simulink model "BEV_Laengsdynamikmodell_v2"  (R2024a)
settings: configuration reference "SharedConfig" (kept outside this file)
values from neighbouring files (symbols this model uses):
  acc_cycle_flag = 0    [simulink_function_handle_v2.m]
  battery = sim_BTMS_interface(battery,config_battery, config_vehicle)    [init_simulation.m]    (also in simulink_function_handle_v2.m = evalin('base', 'battery'))
  config_battery = read_json_config("config/conf_battery.json")    [Sim_v2.m]    (also in init_simulation.m = evalin('base', 'config_battery'); simulink_function_handle_v2.m = cell_loader(config_battery, bat_cell_capacity, bat_celltype )
  config_gearbox = evalin("base", "config_gearbox")    [simulink_function_handle_v2.m]
  config_Inverter = read_json_config("config/conf_Inverter.json")    [Sim_v2.m]
  config_motor = evalin("base","config_motor")    [simulink_function_handle_v2.m]
  config_vehicle = read_json_config(vehicle_config_file)    [Sim_v2.m]    (also in import_dc_cycle.m = evalin('base', 'config_vehicle'); init_simulation.m = evalin('base', 'config_vehicle'); simulink_function_handle_v2.m = evalin('base','config_vehicle'))
  k_FW = 410/(14e3)^2.5    (= 1.76792471652e-08)    [simulink_function_handle_v2.m]
  ModuleType1 = evalin("base","ModuleType1")    [simulink_function_handle_v2.m]
undefined symbols (not defined in the file or in its folder): Analyse, battery_builder_rtmsupport, GB, gcbh, gearbox_map, ModuleAssembly1, motormap
libraries: spsParallelRLCBranchLib x20, nesl_utility x18, GD_Batterymodel_NSGAII_1_lib x12, BatteryProtection x9, spsControlledCurrentSourceLib x8, spsVoltageMeasurementLib x8, fl_lib x7, dspstat3 x4, spsDCVoltageSourceLib x4, spspowerguiLib x4, simulink x3, eePmsmCurrentReferenceGen x2
(part 2 of 5)

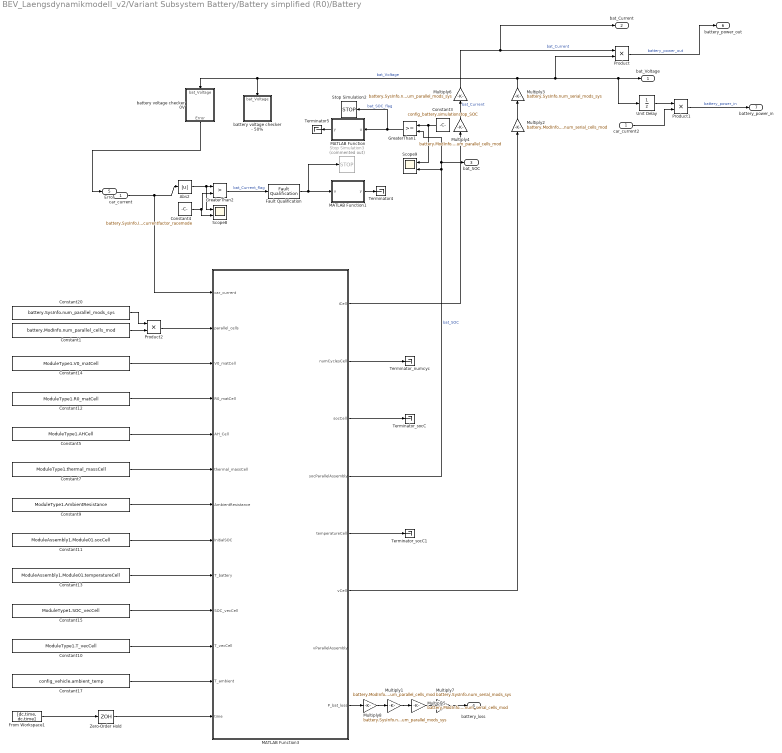
== system BEV_Laengsdynamikmodell_v2/Variant Subsystem Battery/Battery simplified (R0)/Battery ==
  car_current : Inport
  Abs2 : Abs  SaturateOnIntegerOverflow=off
  Constant1 : Constant  Value=battery.ModInfo.num_parallel_cells_mod
  Constant10 : Constant  Value=ModuleType1.T_vecCell
  Constant11 : Constant  Value=ModuleAssembly1.Module01.socCell
  Constant12 : Constant  Value=ModuleType1.R0_matCell
  Constant13 : Constant  Value=ModuleAssembly1.Module01.temperatureCell
  Constant14 : Constant  Value=ModuleType1.V0_matCell
  Constant15 : Constant  Value=ModuleType1.SOC_vecCell
  Constant17 : Constant  Value=config_vehicle.ambient_temp
  Constant20 : Constant  Value=battery.SysInfo.num_parallel_mods_sys
  Constant3 : Constant  Value=config_battery.simulationstop_SOC
  Constant4 : Constant  Value=battery.SysInfo.I_max_sys * config_battery.overcurrentfactor_racemode
  Constant5 : Constant  Value=ModuleType1.AHCell
  Constant7 : Constant  Value=ModuleType1.thermal_massCell
  Constant9 : Constant  Value=ModuleType1.AmbientResistance
  Fault Qualification : BatteryProtection/Fault Qualification  QualTime=3  DisqualTime=6  Ts=-1
      settings: LibrarySourceBlock=batt_sl_lib/Protection/Fault Qualification
  From Workspace1 : FromWorkspace  VariableName=[dc.time, dc.time]
  GreaterThan1 : RelationalOperator  OutDataTypeStr=boolean  RndMeth=Simplest  InputSameDT=off
  GreaterThan2 : RelationalOperator  Operator=>  OutDataTypeStr=boolean  RndMeth=Simplest  InputSameDT=off
  MATLAB Function : MATLAB Function  TreatAsAtomicUnit=on
  MATLAB Function1 : MATLAB Function  TreatAsAtomicUnit=on
  MATLAB Function3 : MATLAB Function  TreatAsAtomicUnit=on
  Multiply1 : Gain  Gain=battery.ModInfo.num_parallel_cells_mod
  Multiply2 : Gain  Gain=battery.ModInfo.num_serial_cells_mod
  Multiply3 : Gain  Gain=battery.SysInfo.num_serial_mods_sys
  Multiply4 : Gain  Gain=battery.ModInfo.num_parallel_cells_mod
  Multiply5 : Gain  Gain=battery.ModInfo.num_serial_cells_mod
  Multiply6 : Gain  Gain=battery.SysInfo.num_parallel_mods_sys
  Multiply7 : Gain  Gain=battery.SysInfo.num_serial_mods_sys
  Multiply8 : Gain  Gain=battery.SysInfo.num_parallel_mods_sys
  Product : Product
  Product1 : Product
  Product2 : Product
  Scope8 : Scope  NumInputPorts=2
  Scope9 : Scope  NumInputPorts=2
  Stop Simulation2 : Stop
  Stop Simulation3 : Stop  Commented=on
  Terminator4 : Terminator
  Terminator5 : Terminator
  Terminator_numcyc : Terminator
  Terminator_socC : Terminator
  Terminator_socC1 : Terminator
  Unit Delay : UnitDelay  SampleTime=-1  HasFrameUpgradeWarning=on
  Zero-Order Hold : ZeroOrderHold  SampleTime=-1
  battery voltage checker - 50% : Subsystem
  battery voltage checker 0V : Subsystem
  car_current2 : InportShadow
  bat_Voltage : Outport
  bat_Current : Outport  Port=2
  bat_SOC : Outport  Port=3
  battery_loss : Outport  Port=4
  Error : Outport  Port=5
  battery_power_out : Outport  Port=6
  battery_power_in : Outport  Port=7
  wires:
  Constant3/1 -> GreaterThan1/1, Scope9/1
  car_current/1 -> MATLAB Function3/1(car_current), Abs2/1
  MATLAB Function3/6(vCell) -> Multiply2/1
  Multiply3/1 -> Product/2, bat_Voltage/1, Unit Delay/1, battery voltage checker - 50%/1(bat_Voltage), battery voltage checker 0V/1(bat_Voltage)  "bat_Voltage"
  Abs2/1 -> Scope8/1, GreaterThan2/1
  Constant4/1 -> Scope8/2, GreaterThan2/2
  MATLAB Function3/4(socParallelAssembly) -> GreaterThan1/2, bat_SOC/1, Scope9/2  "bat_SOC"
  MATLAB Function3/1(iCell) -> Multiply4/1
  GreaterThan1/1 -> Stop Simulation2/1, MATLAB Function/1(u)  "bat_SOC_flag"
  GreaterThan2/1 -> Fault Qualification/1  "bat_Current_flag"
  MATLAB Function/1(y) -> Terminator5/1
  MATLAB Function1/1(y) -> Terminator4/1
  Multiply4/1 -> Multiply6/1  "bat_Current"
  MATLAB Function3/3(socCell) -> Terminator_socC/1
  battery voltage checker 0V/1(Error) -> Error/1
  Multiply2/1 -> Multiply3/1
  Fault Qualification/1 -> Stop Simulation3/1, MATLAB Function1/1(u)
  MATLAB Function3/2(numCyclesCell) -> Terminator_numcyc/1
  MATLAB Function3/5(temperatureCell) -> Terminator_socC1/1
  car_current2/1 -> Product1/2
  Unit Delay/1 -> Product1/1
  Multiply6/1 -> bat_Current/1, Product/1  "bat_Current"
  Product1/1 -> battery_power_in/1  "battery_power_in"
  Product/1 -> battery_power_out/1  "battery_power_out"
  Zero-Order Hold/1 -> MATLAB Function3/13(time)
  From Workspace1/1 -> Zero-Order Hold/1
  Constant5/1 -> MATLAB Function3/5(AH_Cell)
  Constant13/1 -> MATLAB Function3/9(T_battery)
  Constant11/1 -> MATLAB Function3/8(InitialSOC)
  Constant14/1 -> MATLAB Function3/3(V0_matCell)
  Constant12/1 -> MATLAB Function3/4(R0_matCell)
  Constant15/1 -> MATLAB Function3/10(SOC_vecCell)
  Constant7/1 -> MATLAB Function3/6(thermal_massCell)
  Constant10/1 -> MATLAB Function3/11(T_vecCell)
  Constant9/1 -> MATLAB Function3/7(AmbientResistance)
  Constant17/1 -> MATLAB Function3/12(T_ambient)
  Multiply7/1 -> battery_loss/1
  MATLAB Function3/8(P_bat_loss) -> Multiply8/1
  Multiply5/1 -> Multiply7/1
  Multiply1/1 -> Multiply5/1
  Constant1/1 -> Product2/2
  Constant20/1 -> Product2/1
  Product2/1 -> MATLAB Function3/2(parallel_cells)
  Multiply8/1 -> Multiply1/1

== system BEV_Laengsdynamikmodell_v2/Variant Subsystem Gearbox/Gearbox Analytic/Oil Temp ==
  P_V : Inport
  IC : InitialCondition  Value=25
  MATLAB Function : MATLAB Function  TreatAsAtomicUnit=on
  Memory1 : Memory  InitialCondition=config_vehicle.ambient_temp - 273
  Memory2 : Memory  InitialCondition=config_vehicle.ambient_temp - 273
  Scope : Scope
  temp : Outport
  wires:
  MATLAB Function/1(T) -> IC/1  "GB_temp"
  Memory1/1 -> MATLAB Function/1(t)
  P_V/1 -> Memory2/1
  IC/1 -> Scope/1, Memory1/1, temp/1
  Memory2/1 -> MATLAB Function/2(P_V)

== system BEV_Laengsdynamikmodell_v2/Variant Subsystem Gearbox/Gearbox Analytic/Oil Temp Gao ==
  note: entspricht 2pi/60 * 1e-3
  T_wheel : Inport
  rpm_wheel : Inport  Port=2
  MATLAB Function : MATLAB Function  TreatAsAtomicUnit=on
  Memory1 : Memory  InitialCondition=config_vehicle.ambient_temp - 273
  Multiply5 : Gain  Gain=1/9550
  Product2 : Product
  Scope : Scope
  temp : Outport
  wires:
  Product2/1 -> Multiply5/1
  rpm_wheel/1 -> MATLAB Function/3(rpm), Product2/2
  T_wheel/1 -> Product2/1
  MATLAB Function/1(T) -> Scope/1, Memory1/1, temp/1
  Memory1/1 -> MATLAB Function/1(t)
  Multiply5/1 -> MATLAB Function/2(P)

== system BEV_Laengsdynamikmodell_v2/Variant Subsystem Gearbox/Gearbox Analytic/Variant Subsystem Analytic GB ==
  note: 1) Add Subsystem or Model blocks as valid variant choices.
      | 2) You cannot connect blocks at this level. At simulation, connectivity is automatically
      | determined, based on the active variant and port name matching.
  wheel_torque : Inport
  wheel_rpm : Inport  Port=2
  Temp : Inport  Port=3
  Einstufig_Achsparallel : Subsystem  VariantControl=GB_Stufen == 1
  Zweistufig_Achsparallel : Subsystem  VariantControl="GB_Stufen == 2 && GB_Topology == \"achsparallel\""
  Zweistufig_Koaxial : Subsystem  VariantControl="GB_Stufen == 2 && GB_Topology == \"koaxial\""
  P_V : Outport

== system BEV_Laengsdynamikmodell_v2/Variant Subsystem Gearbox/Gearbox Lookup-Table/Oil Temp ==
  P_V : Inport
  IC : InitialCondition  Value=25
  MATLAB Function : MATLAB Function  TreatAsAtomicUnit=on
  Memory1 : Memory  InitialCondition=config_vehicle.ambient_temp - 273
  Memory2 : Memory  InitialCondition=config_vehicle.ambient_temp - 273
  Scope : Scope
  temp : Outport
  wires:
  MATLAB Function/1(T) -> IC/1  "GB_temp"
  Memory1/1 -> MATLAB Function/1(t)
  P_V/1 -> Memory2/1
  IC/1 -> Scope/1, Memory1/1, temp/1
  Memory2/1 -> MATLAB Function/2(P_V)

== system BEV_Laengsdynamikmodell_v2/Variant Subsystem Gearbox/Gearbox Lookup-Table/Oil Temp Gao ==
  note: entspricht 2pi/60 * 1e-3
  T_wheel : Inport
  rpm_wheel : Inport  Port=2
  MATLAB Function : MATLAB Function  TreatAsAtomicUnit=on
  Memory1 : Memory  InitialCondition=config_vehicle.ambient_temp - 273
  Multiply5 : Gain  Gain=1/9550
  Product2 : Product
  Scope : Scope
  temp : Outport
  wires:
  Product2/1 -> Multiply5/1
  rpm_wheel/1 -> MATLAB Function/3(rpm), Product2/2
  T_wheel/1 -> Product2/1
  MATLAB Function/1(T) -> Scope/1, Memory1/1, temp/1
  Memory1/1 -> MATLAB Function/1(t)
  Multiply5/1 -> MATLAB Function/2(P)

== system BEV_Laengsdynamikmodell_v2/Variant Subsystem Gearbox/Gearbox Lookup-Table/Variant Subsystem ==
  note: 1) Add Subsystem or Model blocks as valid variant choices.
      | 2) You cannot connect blocks at this level. At simulation, connectivity is automatically
      | determined, based on the active variant and port name matching.
  wheel_torque : Inport
  wheel_rpm : Inport  Port=2
  Temp : Inport  Port=3
  ETA_map : Subsystem  VariantControl="gearbox_map.map_type == \"Eta\""
  LOSS_map : Subsystem  VariantControl="gearbox_map.map_type == \"Loss\""
  loss_lockup : Outport
  gearbox_efficiency : Outport  Port=2
  gearbox_rpm : Outport  Port=3
  gearbox_torque : Outport  Port=4

== system BEV_Laengsdynamikmodell_v2/Variant Subsystem Inverter/Inverter Analytic/Variant Subsystem ==
  note: 1) Add Subsystem or Model blocks as valid variant choices.
      | 2) You cannot connect blocks at this level. At simulation, connectivity is automatically
      | determined, based on the active variant and port name matching.
  udc : Inport
  rpm : Inport  Port=2
  torque : Inport  Port=3
  terminal_power : Inport  Port=4
  IM_Inverter_IGBT_Analytic : Subsystem  VariantControl=Mode_IM_IGBT
  IM_Inverter_SiC-MOSFET_Analytic : Subsystem  VariantControl=Mode_IM_MOSFET
  PMSM_Inverter_IBGT_Analytic : Subsystem  VariantControl=Mode_PSM_IGBT
  PMSM_Inverter_SiC-MOSFET_Analytic : Subsystem  VariantControl=Mode_PSM_MOSFET
  Conduction_and_Switching_loss : Outport
  idc : Outport  Port=2
  P_inv_total : Outport  Port=3
  P_mot_elec : Outport  Port=4

== system BEV_Laengsdynamikmodell_v2/Variant Subsystem Motor/Motor Analytic/Friction & Windage ==
  note: Gleichung für mechanische Verlustleistung:
      | P_FW = k_FW * n^2.5
  gearbox_rpm : Inport
  Constant : Constant  Value=2.5
  Constant1 : Constant  Value=0
  Constant5 : Constant  Value=k_FW
  Gain : Gain  Gain=2*pi/60
  In2 : InportShadow
  Power : Math  Operator=pow
  Product : Product
  Product2 : Product  Inputs=*/
  Switch : Switch  Criteria=u2 > Threshold  SaturateOnIntegerOverflow=off  InputSameDT=off
  friction torque : Outport
  wires:
  gearbox_rpm/1 -> Power/1  "n_gearbox"
  Constant/1 -> Power/2  "exponent"
  Power/1 -> Product/1
  Constant5/1 -> Product/2
  Product/1 -> Product2/1  "mech powerloss"
  Product2/1 -> Switch/1  "torque"
  In2/1 -> Gain/1  "n_gearbox"
  Gain/1 -> Product2/2, Switch/2
  Switch/1 -> friction torque/1
  Constant1/1 -> Switch/3

== system BEV_Laengsdynamikmodell_v2/Variant Subsystem Motor/Motor Const/Friction & Windage ==
  note: Gleichung für mechanische Verlustleistung:
      | P_FW = k_FW * n^2.5
  gearbox_rpm : Inport
  Constant : Constant  Value=2.5
  Constant1 : Constant  Value=0
  Constant5 : Constant  Value=k_FW
  Gain : Gain  Gain=2*pi/60
  In2 : InportShadow
  Power : Math  Operator=pow
  Product : Product
  Product2 : Product  Inputs=*/
  Switch : Switch  Criteria=u2 > Threshold  SaturateOnIntegerOverflow=off  InputSameDT=off
  friction torque : Outport
  wires:
  gearbox_rpm/1 -> Power/1  "n_gearbox"
  Constant/1 -> Power/2  "exponent"
  Power/1 -> Product/1
  Constant5/1 -> Product/2
  Product/1 -> Product2/1  "mech powerloss"
  Product2/1 -> Switch/1  "torque"
  In2/1 -> Gain/1  "n_gearbox"
  Gain/1 -> Product2/2, Switch/2
  Switch/1 -> friction torque/1
  Constant1/1 -> Switch/3

== system BEV_Laengsdynamikmodell_v2/Variant Subsystem Motor/Motor Lookup-Table/Friction & Windage ==
  note: Gleichung für mechanische Verlustleistung:
      | P_FW = k_FW * n^2.5
  gearbox_rpm : Inport
  Constant : Constant  Value=2.5
  Constant1 : Constant  Value=0
  Constant5 : Constant  Value=k_FW
  Gain : Gain  Gain=2*pi/60
  In2 : InportShadow
  Power : Math  Operator=pow
  Product : Product
  Product2 : Product  Inputs=*/
  Switch : Switch  Criteria=u2 > Threshold  SaturateOnIntegerOverflow=off  InputSameDT=off
  friction torque : Outport
  wires:
  gearbox_rpm/1 -> Power/1  "n_gearbox"
  Constant/1 -> Power/2  "exponent"
  Power/1 -> Product/1
  Constant5/1 -> Product/2
  Product/1 -> Product2/1  "mech powerloss"
  Product2/1 -> Switch/1  "torque"
  In2/1 -> Gain/1  "n_gearbox"
  Gain/1 -> Product2/2, Switch/2
  Switch/1 -> friction torque/1
  Constant1/1 -> Switch/3

== system BEV_Laengsdynamikmodell_v2/Variant Subsystem Battery/Battery Analytic (RC3)/Battery/battery voltage checker - 50% ==
  bat_Voltage : Inport
  Constant : Constant  Value=acc_cycle_flag
  Constant5 : Constant  Value=0.5 * battery.SysInfo.U_max_sys
  Data Type Conversion : DataTypeConversion  OutDataTypeStr=double  SaturateOnIntegerOverflow=off  RndMeth=Floor
  Fault Qualification : BatteryProtection/Fault Qualification  QualTime=2  DisqualTime=4  Ts=-1
      settings: LibrarySourceBlock=batt_sl_lib/Protection/Fault Qualification
  GreaterThan3 : RelationalOperator  Operator=>  OutDataTypeStr=boolean  RndMeth=Simplest  InputSameDT=off
  MATLAB Function2 : MATLAB Function  TreatAsAtomicUnit=on
  Stop Simulation : Stop
  Unit Delay : UnitDelay  SampleTime=-1  HasFrameUpgradeWarning=on
  wires:
  Constant/1 -> MATLAB Function2/3(z)
  Fault Qualification/1 -> MATLAB Function2/1(u)
  MATLAB Function2/2(st) -> Stop Simulation/1
  Data Type Conversion/1 -> MATLAB Function2/2(d)
  Unit Delay/1 -> Data Type Conversion/1
  MATLAB Function2/1(y) -> Unit Delay/1
  bat_Voltage/1 -> GreaterThan3/2
  GreaterThan3/1 -> Fault Qualification/1
  Constant5/1 -> GreaterThan3/1

== system BEV_Laengsdynamikmodell_v2/Variant Subsystem Battery/Battery Analytic (RC3)/Battery/battery voltage checker 0V ==
  bat_Voltage : Inport
  Constant7 : Constant  Value=0
  Fault Qualification1 : BatteryProtection/Fault Qualification  QualTime=1  DisqualTime=3  Ts=-1
      settings: LibrarySourceBlock=batt_sl_lib/Protection/Fault Qualification
  GreaterThan4 : RelationalOperator  Operator=>  OutDataTypeStr=boolean  RndMeth=Simplest  InputSameDT=off
  Error : Outport
  wires:
  Fault Qualification1/1 -> Error/1
  bat_Voltage/1 -> GreaterThan4/2
  GreaterThan4/1 -> Fault Qualification1/1
  Constant7/1 -> GreaterThan4/1

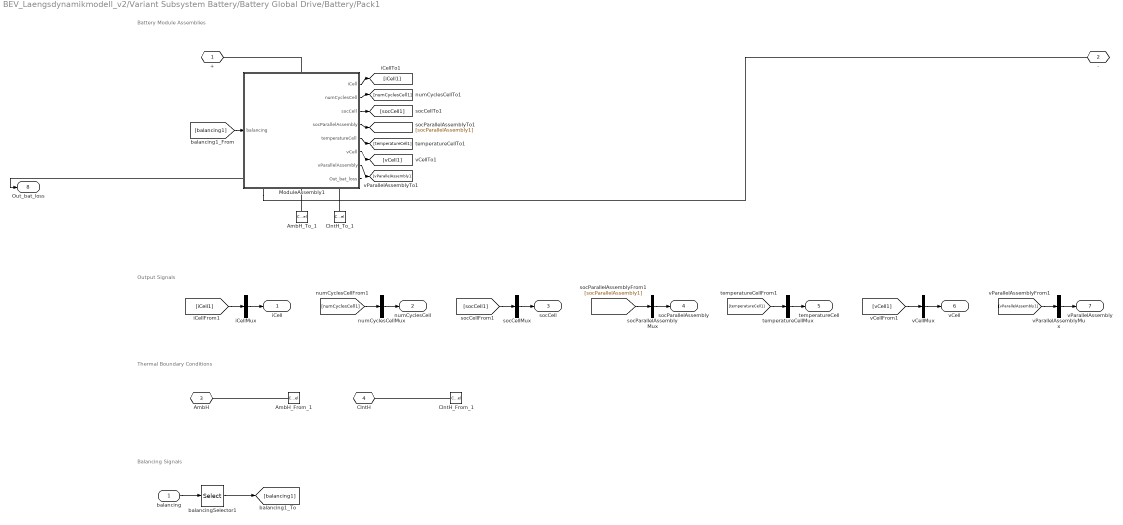
== system BEV_Laengsdynamikmodell_v2/Variant Subsystem Battery/Battery Global Drive/Battery/Pack1 ==
  note: Balancing Signals
  note: Thermal Boundary Conditions
  note: Output Signals
  note: Battery Module Assemblies
  balancing : Inport  PortDimensions=120
  AmbH_From_1 : ConnectionLabel  Label=ambH_1
  AmbH_To_1 : ConnectionLabel  Label=ambH_1
  ClntH_From_1 : ConnectionLabel  Label=clntH_1
  ClntH_To_1 : ConnectionLabel  Label=clntH_1
  ModuleAssembly1 : Subsystem  LoadFcn=battery_builder_rtmsupport('loadfcn',gcbh);
      settings: CopyFcn=battery_builder_rtmsupport('copyfcn',gcbh);  PreCopyFcn=battery_builder_rtmsupport('precopyfcn',gcbh);  PreDeleteFcn=battery_builder_rtmsupport('predeletefcn',gcbh);  PortSchema="{\"entries\":[{\"content\":{\"sides\":[{\"content\":{\"connectorIds\":[\"LConn1\"]},\"type\":\"ConnectorPlacement.EquallySpacedRectSide\",\"uuid\":\"39e93321-efac-446f-a75c-eda4d8d6b0d6\"},{\"content\":{\"connectorIds\":[\"RConn1\",\"RConn2\",\"RConn3\"],\"side\":\"RIGHT\"},\"type\":\"ConnectorPlacement.EquallySpacedRectSide\",\"uuid\":\"10ad7812-c6c9-4cb3-b6be-c67a3fc87af4\"},{\"content\":{\"connectorIds\":[\"In1\"],\"side\":\"TOP\"},\"type\":\"ConnectorPlacement.EquallySpacedRectSide\",\"uuid\":\"ea32dac7-a4ac-4f16-bcf8-bfac99073aa1\"},{\"content\":{\"connectorIds\":[\"Out1\",\"Out2\",\"Out3\",\"Out4\",\"Out5\",\"Out6\",\"Out7\",\"Out8\"],\"side\":\"BOTTOM\"},\"type\":\"ConnectorPlacement.EquallySpacedRectSide\",\"uuid\":\"2a45af1c-2d64-4e86-8177-57e80a443e25\"}]},\"type\":\"ConnectorPlacement.EquallySpacedConnector\",\"uuid\":\"ff988f0c-c525-4dd2-8156-8cb001cdab44\"}],\"packageUris\":[\"http://schema.mathworks.com/mf0/Connector/R2020b\"],\"version\":\"1.0\"}"
      mask Display: image('$imagefile')
  balancingSelector1 : Selector  InputPortWidth=120  IndexOptions=Index vector (dialog)  Indices="[1    2    3    4    5    6    7    8    9   10   11   12   13   14   15   16   17   18   19   20   21   22   23   24   25   26   27   28   29   30   31   32   33   34   35   36   37   38   39   40   41   42   43   44   45   46   47   48   49   50   51   52   53   54   55   56   57   58   59   60   61   62   63   64   65   66   67   68   69   70   71   72   73   74   75   76   77   78   79   80   81   82   83   84   85   86   87   88   89   90   91   92   93   94   95   96   97   98   99  100  101  102  103  104  105  106  107  108  109  110  111  112  113  114  115  116  117  118  119  120]"  OutputSizes=1
  iCellMux : Mux  Inputs=1
  numCyclesCellMux : Mux  Inputs=1
  socCellMux : Mux  Inputs=1
  socParallelAssemblyMux : Mux  Inputs=1
  temperatureCellMux : Mux  Inputs=1
  vCellMux : Mux  Inputs=1
  vParallelAssemblyMux : Mux  Inputs=1
  + : PMIOPort  Side=Left
  - : PMIOPort  Port=2  Side=Right
  AmbH : PMIOPort  Port=3  Side=Right  ConnectionType=Connection: foundation.thermal.thermal
  ClntH : PMIOPort  Port=4  Side=Right  ConnectionType=Connection: foundation.thermal.thermal
  iCell : Outport
  numCyclesCell : Outport  Port=2
  socCell : Outport  Port=3
  socParallelAssembly : Outport  Port=4
  temperatureCell : Outport  Port=5
  vCell : Outport  Port=6
  vParallelAssembly : Outport  Port=7
  Out_bat_loss : Outport  Port=8
  wires:
  balancingSelector1/1 -> [balancing1]
  balancing/1 -> balancingSelector1/1
  [balancing1] -> ModuleAssembly1/1(balancing)
  [vParallelAssembly1] -> vParallelAssemblyMux/1
  vParallelAssemblyMux/1 -> vParallelAssembly/1
  ModuleAssembly1/7(vParallelAssembly) -> [vParallelAssembly1]
  [vCell1] -> vCellMux/1
  vCellMux/1 -> vCell/1
  ModuleAssembly1/6(vCell) -> [vCell1]
  [temperatureCell1] -> temperatureCellMux/1
  temperatureCellMux/1 -> temperatureCell/1
  ModuleAssembly1/5(temperatureCell) -> [temperatureCell1]
  [socParallelAssembly1] -> socParallelAssemblyMux/1
  socParallelAssemblyMux/1 -> socParallelAssembly/1
  ModuleAssembly1/4(socParallelAssembly) -> [socParallelAssembly1]
  [socCell1] -> socCellMux/1
  socCellMux/1 -> socCell/1
  ModuleAssembly1/3(socCell) -> [socCell1]
  [numCyclesCell1] -> numCyclesCellMux/1
  numCyclesCellMux/1 -> numCyclesCell/1
  ModuleAssembly1/2(numCyclesCell) -> [numCyclesCell1]
  [iCell1] -> iCellMux/1
  iCellMux/1 -> iCell/1
  ModuleAssembly1/1(iCell) -> [iCell1]
  ModuleAssembly1/8(Out_bat_loss) -> Out_bat_loss/1
  connections:
  ClntH_From_1/LConn1 -- ClntH/RConn1
  ClntH_To_1/LConn1 -- ModuleAssembly1/RConn3
  AmbH_From_1/LConn1 -- AmbH/RConn1
  AmbH_To_1/LConn1 -- ModuleAssembly1/RConn2
  ModuleAssembly1/RConn1 -- -/RConn1
  ModuleAssembly1/LConn1 -- +/RConn1

== system BEV_Laengsdynamikmodell_v2/Variant Subsystem Battery/Battery Global Drive/Battery/battery voltage checker - 50% ==
  bat_Voltage : Inport
  Constant : Constant  Value=acc_cycle_flag
  Constant5 : Constant  Value=0.5 * battery.SysInfo.U_max_sys
  Data Type Conversion : DataTypeConversion  OutDataTypeStr=double  SaturateOnIntegerOverflow=off  RndMeth=Floor
  Fault Qualification : BatteryProtection/Fault Qualification  QualTime=2  DisqualTime=4  Ts=-1
      settings: LibrarySourceBlock=batt_sl_lib/Protection/Fault Qualification
  GreaterThan3 : RelationalOperator  Operator=>  OutDataTypeStr=boolean  RndMeth=Simplest  InputSameDT=off
  MATLAB Function2 : MATLAB Function  TreatAsAtomicUnit=on
  Stop Simulation : Stop
  Unit Delay : UnitDelay  SampleTime=-1  HasFrameUpgradeWarning=on
  wires:
  Constant5/1 -> GreaterThan3/1
  GreaterThan3/1 -> Fault Qualification/1
  bat_Voltage/1 -> GreaterThan3/2
  MATLAB Function2/1(y) -> Unit Delay/1
  Unit Delay/1 -> Data Type Conversion/1
  Data Type Conversion/1 -> MATLAB Function2/2(d)
  MATLAB Function2/2(st) -> Stop Simulation/1
  Fault Qualification/1 -> MATLAB Function2/1(u)
  Constant/1 -> MATLAB Function2/3(z)

== system BEV_Laengsdynamikmodell_v2/Variant Subsystem Battery/Battery Global Drive/Battery/battery voltage checker 0V ==
  bat_Voltage : Inport
  Constant7 : Constant  Value=0
  Fault Qualification1 : BatteryProtection/Fault Qualification  QualTime=1  DisqualTime=3  Ts=-1
      settings: LibrarySourceBlock=batt_sl_lib/Protection/Fault Qualification
  GreaterThan4 : RelationalOperator  Operator=>  OutDataTypeStr=boolean  RndMeth=Simplest  InputSameDT=off
  Error : Outport
  wires:
  Constant7/1 -> GreaterThan4/1
  GreaterThan4/1 -> Fault Qualification1/1
  bat_Voltage/1 -> GreaterThan4/2
  Fault Qualification1/1 -> Error/1

== system BEV_Laengsdynamikmodell_v2/Variant Subsystem Battery/Battery simplified (R0)/Battery/battery voltage checker - 50% ==
  bat_Voltage : Inport
  Constant : Constant  Value=acc_cycle_flag
  Constant5 : Constant  Value=0.5 * battery.SysInfo.U_max_sys
  Data Type Conversion : DataTypeConversion  OutDataTypeStr=double  SaturateOnIntegerOverflow=off  RndMeth=Floor
  Fault Qualification : BatteryProtection/Fault Qualification  QualTime=2  DisqualTime=4  Ts=-1
      settings: LibrarySourceBlock=batt_sl_lib/Protection/Fault Qualification
  GreaterThan3 : RelationalOperator  Operator=>  OutDataTypeStr=boolean  RndMeth=Simplest  InputSameDT=off
  MATLAB Function2 : MATLAB Function  TreatAsAtomicUnit=on
  Stop Simulation : Stop
  Unit Delay : UnitDelay  SampleTime=-1  HasFrameUpgradeWarning=on
  wires:
  Constant5/1 -> GreaterThan3/1
  GreaterThan3/1 -> Fault Qualification/1
  bat_Voltage/1 -> GreaterThan3/2
  MATLAB Function2/1(y) -> Unit Delay/1
  Unit Delay/1 -> Data Type Conversion/1
  Data Type Conversion/1 -> MATLAB Function2/2(d)
  MATLAB Function2/2(st) -> Stop Simulation/1
  Fault Qualification/1 -> MATLAB Function2/1(u)
  Constant/1 -> MATLAB Function2/3(z)

== system BEV_Laengsdynamikmodell_v2/Variant Subsystem Battery/Battery simplified (R0)/Battery/battery voltage checker 0V ==
  bat_Voltage : Inport
  Constant7 : Constant  Value=0
  Fault Qualification1 : BatteryProtection/Fault Qualification  QualTime=1  DisqualTime=3  Ts=-1
      settings: LibrarySourceBlock=batt_sl_lib/Protection/Fault Qualification
  GreaterThan4 : RelationalOperator  Operator=>  OutDataTypeStr=boolean  RndMeth=Simplest  InputSameDT=off
  Error : Outport
  wires:
  Constant7/1 -> GreaterThan4/1
  GreaterThan4/1 -> Fault Qualification1/1
  bat_Voltage/1 -> GreaterThan4/2
  Fault Qualification1/1 -> Error/1

== system BEV_Laengsdynamikmodell_v2/Variant Subsystem Gearbox/Gearbox Analytic/Variant Subsystem Analytic GB/Einstufig_Achsparallel ==
  wheel_torque : Inport
  wheel_rpm : Inport  Port=2
  Temp : Inport  Port=3
  Add : Sum
  MATLAB Function : MATLAB Function  TreatAsAtomicUnit=on
  Ölpumpe : Subsystem
  P_V : Outport
  wires:
  wheel_rpm/1 -> Ölpumpe/1(nrad), MATLAB Function/2(nrad)
  MATLAB Function/1(P_V) -> Add/1
  wheel_torque/1 -> MATLAB Function/1(Mrad)
  Temp/1 -> MATLAB Function/3(Temp)
  Add/1 -> P_V/1
  Ölpumpe/1(power_oilpump) -> Add/2

== system BEV_Laengsdynamikmodell_v2/Variant Subsystem Gearbox/Gearbox Analytic/Variant Subsystem Analytic GB/Zweistufig_Achsparallel ==
  wheel_torque : Inport
  wheel_rpm : Inport  Port=2
  Temp : Inport  Port=3
  Add : Sum
  MATLAB Function : MATLAB Function  TreatAsAtomicUnit=on
  Ölpumpe : Subsystem
  P_V : Outport
  wires:
  wheel_rpm/1 -> Ölpumpe/1(nrad), MATLAB Function/2(nrad)
  MATLAB Function/1(P_V) -> Add/1
  wheel_torque/1 -> MATLAB Function/1(Mrad)
  Temp/1 -> MATLAB Function/3(Temp)
  Add/1 -> P_V/1
  Ölpumpe/1(power_oilpump) -> Add/2

== system BEV_Laengsdynamikmodell_v2/Variant Subsystem Gearbox/Gearbox Analytic/Variant Subsystem Analytic GB/Zweistufig_Koaxial ==
  wheel_torque : Inport
  wheel_rpm : Inport  Port=2
  Temp : Inport  Port=3
  Add : Sum
  MATLAB Function : MATLAB Function  TreatAsAtomicUnit=on
  Ölpumpe : Subsystem
  P_V : Outport
  wires:
  Temp/1 -> MATLAB Function/3(Temp)
  wheel_torque/1 -> MATLAB Function/1(Mrad)
  MATLAB Function/1(P_V) -> Add/1
  wheel_rpm/1 -> Ölpumpe/1(nrad), MATLAB Function/2(nrad)
  Add/1 -> P_V/1
  Ölpumpe/1(power_oilpump) -> Add/2

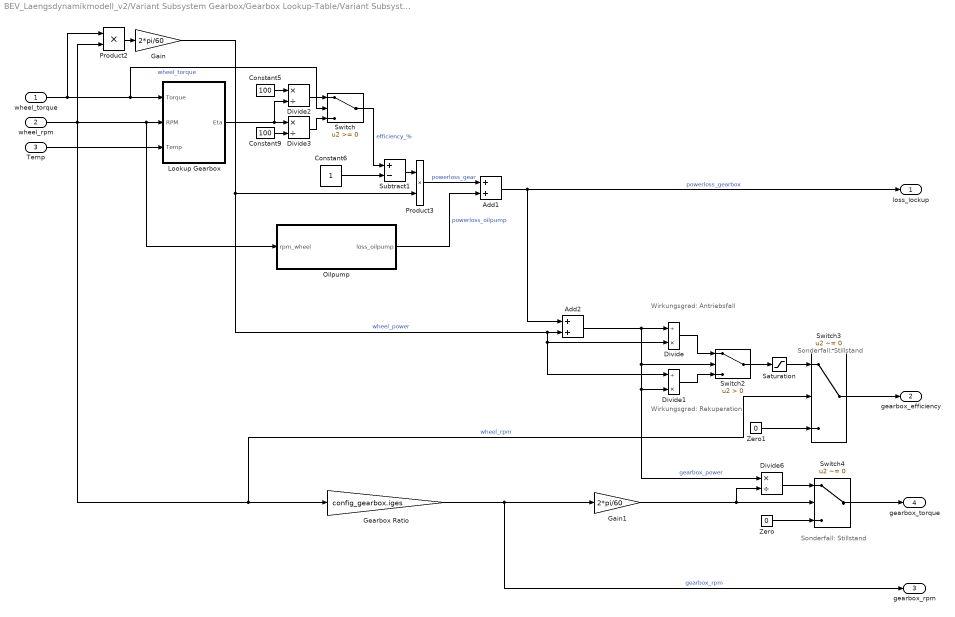
== system BEV_Laengsdynamikmodell_v2/Variant Subsystem Gearbox/Gearbox Lookup-Table/Variant Subsystem/ETA_map ==
  note: Sonderfall: Stillstand
  note: Sonderfall: Stillstand
  note: Wirkungsgrad:
      | Antriebsfall
  note: Wirkungsgrad:
      | Rekuperation
  wheel_torque : Inport
  wheel_rpm : Inport  Port=2
  Temp : Inport  Port=3
  Add1 : Sum
  Add2 : Sum
  Constant5 : Constant  Value=100
  Constant6 : Constant
  Constant9 : Constant  Value=100
  Divide : Product  Inputs=/*
  Divide1 : Product  Inputs=/*
  Divide2 : Product  Inputs=*/
  Divide3 : Product  Inputs=*/
  Divide6 : Product  Inputs=*/
  Gain : Gain  Gain=2*pi/60
  Gain1 : Gain  Gain=2*pi/60
  Gearbox Ratio : Gain  Gain=config_gearbox.iges
  Lookup Gearbox : Subsystem  Variant=on
  Oilpump : Subsystem
  Product2 : Product  Inputs=**
  Product3 : Product  Inputs=**
  Saturation : Saturate  UpperLimit=inf  LowerLimit=0
  Subtract1 : Sum  Inputs=+-
  Switch : Switch  SaturateOnIntegerOverflow=off  InputSameDT=off
  Switch2 : Switch  Criteria=u2 > Threshold  SaturateOnIntegerOverflow=off  InputSameDT=off
  Switch3 : Switch  Criteria=u2 ~= 0  SaturateOnIntegerOverflow=off  InputSameDT=off
  Switch4 : Switch  Criteria=u2 ~= 0  SaturateOnIntegerOverflow=off  InputSameDT=off
  Zero : Constant  Value=0  OutDataTypeStr=Inherit: Inherit via back propagation
  Zero1 : Constant  Value=0  OutDataTypeStr=Inherit: Inherit via back propagation
  loss_lockup : Outport
  gearbox_efficiency : Outport  Port=2
  gearbox_rpm : Outport  Port=3
  gearbox_torque : Outport  Port=4
  wires:
  wheel_torque/1 -> Lookup Gearbox/1(Torque), Switch/2, Product2/1  "wheel_torque"
  Divide1/1 -> Switch2/3
  Product2/1 -> Gain/1
  wheel_rpm/1 -> Switch3/2, Gearbox Ratio/1, Product2/2, Oilpump/1(rpm_wheel), Lookup Gearbox/2(RPM)  "wheel_rpm"
  Constant6/1 -> Subtract1/2
  Subtract1/1 -> Product3/1
  Switch/1 -> Subtract1/1  "efficiency_%"
  Product3/1 -> Add1/1  "powerloss_gear"
  Zero1/1 -> Switch3/3
  Switch2/1 -> Saturation/1
  Divide2/1 -> Switch/1
  Zero/1 -> Switch4/3
  Switch4/1 -> gearbox_torque/1
  Switch3/1 -> gearbox_efficiency/1
  Divide6/1 -> Switch4/1
  Gearbox Ratio/1 -> Gain1/1, gearbox_rpm/1  "gearbox_rpm"
  Divide3/1 -> Switch/3
  Add2/1 -> Switch2/2, Divide6/1, Divide1/2, Divide/1  "gearbox_power"
  Gain1/1 -> Switch4/2, Divide6/2
  Temp/1 -> Lookup Gearbox/3(Temp)
  Gain/1 -> Product3/2, Divide1/1, Divide/2, Add2/2  "wheel_power"
  Add1/1 -> Add2/1, loss_lockup/1  "powerloss_gearbox"
  Constant9/1 -> Divide3/2
  Oilpump/1(loss_oilpump) -> Add1/2  "powerloss_oilpump"
  Lookup Gearbox/1(Eta) -> Divide2/2, Divide3/1
  Divide/1 -> Switch2/1
  Constant5/1 -> Divide2/1
  Saturation/1 -> Switch3/1

== system BEV_Laengsdynamikmodell_v2/Variant Subsystem Gearbox/Gearbox Lookup-Table/Variant Subsystem/LOSS_map ==
  note: Sonderfall: Stillstand
  note: Wirkungsgrad: Antriebsfall
  note: Wirkungsgrad: Rekuperation
  note: Sonderfall: Stillstand
  wheel_torque : Inport
  wheel_rpm : Inport  Port=2
  Temp : Inport  Port=3
  Add1 : Sum
  Add2 : Sum
  Divide : Product  Inputs=/*
  Divide1 : Product  Inputs=/*
  Divide6 : Product  Inputs=*/
  Gain : Gain  Gain=2*pi/60
  Gain1 : Gain  Gain=2*pi/60
  Gearbox Ratio : Gain  Gain=config_gearbox.iges
  Lookup Gearbox : Subsystem  Variant=on
  Oilpump : Subsystem
  Product2 : Product  Inputs=**
  Saturation : Saturate  UpperLimit=inf  LowerLimit=0
  Switch2 : Switch  Criteria=u2 > Threshold  SaturateOnIntegerOverflow=off  InputSameDT=off
  Switch3 : Switch  Criteria=u2 ~= 0  SaturateOnIntegerOverflow=off  InputSameDT=off
  Switch4 : Switch  Criteria=u2 ~= 0  SaturateOnIntegerOverflow=off  InputSameDT=off
  Zero : Constant  Value=0  OutDataTypeStr=Inherit: Inherit via back propagation
  Zero1 : Constant  Value=0  OutDataTypeStr=Inherit: Inherit via back propagation
  loss_lockup : Outport
  gearbox_efficiency : Outport  Port=2
  gearbox_rpm : Outport  Port=3
  gearbox_torque : Outport  Port=4
  wires:
  Gain/1 -> Divide1/1, Divide/2, Add2/2  "wheel_power"
  wheel_torque/1 -> Lookup Gearbox/1(Torque), Product2/1  "wheel_torque"
  Lookup Gearbox/1(Loss) -> Add1/1  "powerloss_gear"
  Product2/1 -> Gain/1
  Switch4/1 -> gearbox_torque/1
  Switch3/1 -> gearbox_efficiency/1
  Gearbox Ratio/1 -> gearbox_rpm/1, Gain1/1  "gearbox_rpm"
  Switch2/1 -> Saturation/1
  Divide/1 -> Switch2/1
  Add2/1 -> Divide/1, Switch2/2, Divide1/2, Divide6/1  "gearbox_power"
  Zero/1 -> Switch4/3
  Divide6/1 -> Switch4/1
  Divide1/1 -> Switch2/3
  Oilpump/1(loss_oilpump) -> Add1/2  "powerloss_oilpump"
  Add1/1 -> loss_lockup/1, Add2/1  "powerloss_gearbox"
  Temp/1 -> Lookup Gearbox/3(Temp)
  Gain1/1 -> Switch4/2, Divide6/2
  wheel_rpm/1 -> Switch3/2, Gearbox Ratio/1, Product2/2, Lookup Gearbox/2(RPM), Oilpump/1(rpm_wheel)  "wheel_rpm"
  Zero1/1 -> Switch3/3
  Saturation/1 -> Switch3/1

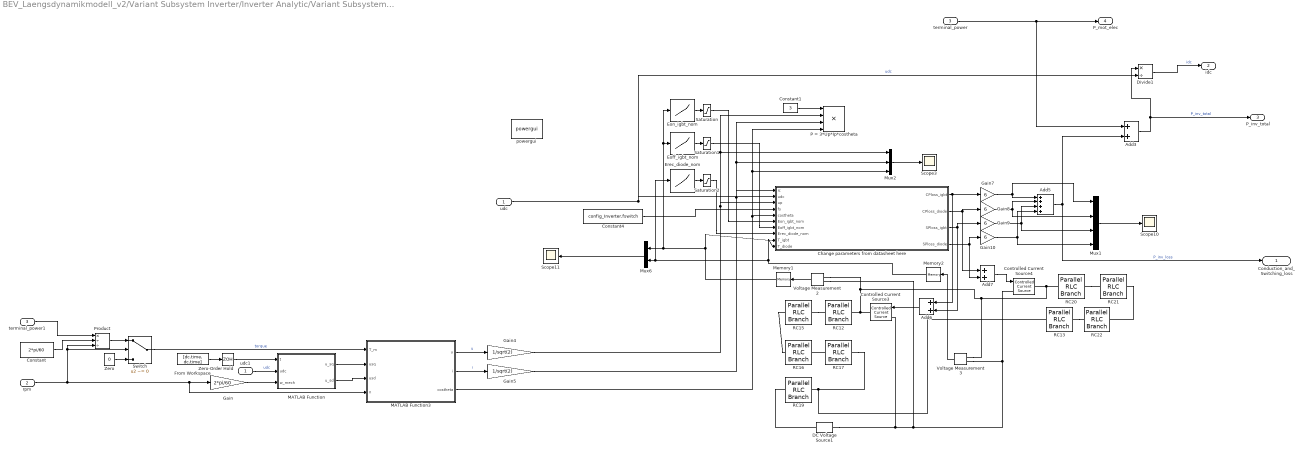
== system BEV_Laengsdynamikmodell_v2/Variant Subsystem Inverter/Inverter Analytic/Variant Subsystem/IM_Inverter_IGBT_Analytic ==
  udc : Inport
  rpm : Inport  Port=2
  terminal_power : Inport  Port=3
  Add3 : Sum
  Add5 : Sum  Inputs=++++
  Add6 : Sum
  Add7 : Sum
  Change parameters from datasheet here : MATLAB Function  TreatAsAtomicUnit=on
  Constant : Constant  Value=2*pi/60
  Constant1 : Constant  Value=3
  Constant4 : Constant  Value=config_Inverter.fswitch
  Controlled Current Source3 : spsControlledCurrentSourceLib/Controlled Current Source  Initialize=on  Source_Type=AC  Amplitude=0  Phase=0  Frequency=0  Measurements=None
  Controlled Current Source4 : spsControlledCurrentSourceLib/Controlled Current Source  Initialize=on  Source_Type=AC  Amplitude=0  Phase=0  Frequency=0  Measurements=None
  DC Voltage Source1 : spsDCVoltageSourceLib/DC Voltage Source  Amplitude=25  Measurements=None
  Divide1 : Product  Inputs=*/
  Eoff_igbt_nom : Lookup_n-D  NumberOfTableDimensions=1  BreakpointsForDimension1=[25, 150, 175]  Table="[23.5*1e-3,  29*1e-3,  30*1e-3]"  InternalRulePriority=Speed  RndMeth=Simplest
  Eon_igbt_nom : Lookup_n-D  NumberOfTableDimensions=1  BreakpointsForDimension1=[25, 150, 175]  Table="[13.5*1e-3,  17.5*1e-3,  18*1e-3]"  InternalRulePriority=Speed  RndMeth=Simplest
  Erec_diode_nom : Lookup_n-D  NumberOfTableDimensions=1  BreakpointsForDimension1=[25, 150, 175]  Table="[7*1e-3,  13*1e-3,  15*1e-3]"  InternalRulePriority=Speed  RndMeth=Simplest
  From Workspace : FromWorkspace  VariableName=[dc.time, dc.time]
  Gain : Gain  Gain=2*pi/60
  Gain{7..10} (4 alike) : Gain  Gain=6
  Gain4 : Gain  Gain=1/sqrt(2)
  Gain5 : Gain  Gain=1/sqrt(2)
  MATLAB Function : MATLAB Function  TreatAsAtomicUnit=on
  MATLAB Function3 : MATLAB Function  TreatAsAtomicUnit=on
  Memory1 : Memory  InitialCondition=25  InheritSampleTime=on
  Memory2 : Memory  InitialCondition=25  InheritSampleTime=on
  Mux1 : Mux
  Mux2 : Mux  Inputs=3
  Mux6 : Mux  Inputs=2
  P = 3*Up*Ip*costheta : Product  Inputs=4
  Product : Product  Inputs=*//
  RC12 : spsParallelRLCBranchLib/Parallel RLC Branch  LConnTagsString=a  RConnTagsString=__new0  BranchType=RC  Resistance=config_Inverter.R1igbt  Inductance=1e-3  SetiL0=off  InitialCurrent=0  Capacitance=config_Inverter.C1igbt  Setx0=off  InitialVoltage=0  Measurements=None
  RC13 : spsParallelRLCBranchLib/Parallel RLC Branch  LConnTagsString=a  RConnTagsString=__new0  BranchType=RC  Resistance=config_Inverter.R4diode  Inductance=1e-3  SetiL0=off  InitialCurrent=0  Capacitance=config_Inverter.C4diode  Setx0=off  InitialVoltage=0  Measurements=None
  RC15 : spsParallelRLCBranchLib/Parallel RLC Branch  LConnTagsString=a  RConnTagsString=__new0  BranchType=RC  Resistance=config_Inverter.R2igbt  Inductance=1e-3  SetiL0=off  InitialCurrent=0  Capacitance=config_Inverter.C2igbt  Setx0=off  InitialVoltage=0  Measurements=None
  RC16 : spsParallelRLCBranchLib/Parallel RLC Branch  LConnTagsString=a  RConnTagsString=__new0  BranchType=RC  Resistance=config_Inverter.R3igbt  Inductance=1e-3  SetiL0=off  InitialCurrent=0  Capacitance=config_Inverter.C3igbt  Setx0=off  InitialVoltage=0  Measurements=None
  RC17 : spsParallelRLCBranchLib/Parallel RLC Branch  LConnTagsString=a  RConnTagsString=__new0  BranchType=RC  Resistance=config_Inverter.R4igbt  Inductance=1e-3  SetiL0=off  InitialCurrent=0  Capacitance=config_Inverter.C4igbt  Setx0=off  InitialVoltage=0  Measurements=None
  RC19 : spsParallelRLCBranchLib/Parallel RLC Branch  LConnTagsString=a  RConnTagsString=__new0  BranchType=R  Resistance=config_Inverter.R6igbt  Inductance=1e-3  SetiL0=off  InitialCurrent=0  Capacitance=175  Setx0=on  InitialVoltage=0  Measurements=None
  RC20 : spsParallelRLCBranchLib/Parallel RLC Branch  LConnTagsString=a  RConnTagsString=__new0  BranchType=RC  Resistance=config_Inverter.R1diode  Inductance=1e-3  SetiL0=off  InitialCurrent=0  Capacitance=config_Inverter.C1diode  Setx0=off  InitialVoltage=0  Measurements=None
  RC21 : spsParallelRLCBranchLib/Parallel RLC Branch  LConnTagsString=a  RConnTagsString=__new0  BranchType=RC  Resistance=config_Inverter.R2diode  Inductance=1e-3  SetiL0=off  InitialCurrent=0  Capacitance=config_Inverter.C2diode  Setx0=off  InitialVoltage=0  Measurements=None
  RC22 : spsParallelRLCBranchLib/Parallel RLC Branch  LConnTagsString=a  RConnTagsString=__new0  BranchType=RC  Resistance=config_Inverter.R3diode  Inductance=1e-3  SetiL0=off  InitialCurrent=0  Capacitance=config_Inverter.C3diode  Setx0=off  InitialVoltage=0  Measurements=None
  Saturation : Saturate  UpperLimit=18*1e-3  LowerLimit=13.5*1e-3
  Saturation1 : Saturate  UpperLimit=30*1e-3  LowerLimit=23.5*1e-3
  Saturation2 : Saturate  UpperLimit=15*1e-3  LowerLimit=7*1e-3
  Scope10 : Scope
  Scope11 : Scope
  Scope3 : Scope
  Switch : Switch  Criteria=u2 ~= 0  SaturateOnIntegerOverflow=off  InputSameDT=off
  Voltage Measurement2 : spsVoltageMeasurementLib/Voltage Measurement  PhasorSimulation=off  OutputType=Complex  PSBequivalent=0
  Voltage Measurement3 : spsVoltageMeasurementLib/Voltage Measurement  PhasorSimulation=off  OutputType=Complex  PSBequivalent=0
  Zero : Constant  Value=0  OutDataTypeStr=Inherit: Inherit via back propagation
  Zero-Order Hold : ZeroOrderHold  SampleTime=-1
  powergui : spspowerguiLib/powergui  Priority=1  SimulationMode=Discrete  SampleTime=1  frequency=60  Iterations=50  frequencyindice=0  Pbase=100e6  ErrMax=1e-4  UnitsV=kV  UnitsW=MW  buscounter=0  FunctionMessages=on  echomessages=on  EnableUseOfTLC=off  CurrentSourceSwitches=off  DisableSnubberDevices=off  DisableRonSwitches=off  DisableVfSwitches=off  DisplayEquations=off  AutomaticDiscreteSolvers=off  SolverType=Backward Euler  Interpol=off  ExternalGateDelay=off  methode=off  Ts=100  x0status=blocks  SPID=off  SwTol=0  HookPort=off  NonlinearTolerance=1e-4  nMaxIteration=100  ContinueOnMaxIteration=off  RestoreLinks=warning  ResistiveCurrentMeasurement=off  Frange=[0:2:500]  Ylog=off  Xlog=on  ShowGrid=off  save=off  variable=ZData  structure=0  ZoomFFT=off  StartTime=0.0  cycles=1  DisplayStyle=1  fundamental=60  FreqAxis=off  MaxFrequency=1000  frequencyindicesteady=1  RmsSteady=1  display=off
  terminal_power1 : InportShadow  Port=3
  udc1 : InportShadow
  Conduction_and_Switching_loss : Outport
  idc : Outport  Port=2
  P_inv_total : Outport  Port=3
  P_mot_elec : Outport  Port=4
  wires:
  Eon_igbt_nom/1 -> Saturation/1
  Erec_diode_nom/1 -> Saturation2/1
  Eoff_igbt_nom/1 -> Saturation1/1
  Gain4/1 -> Change parameters from datasheet here/3(up), Mux2/1, P = 3*Up*Ip*costheta/2
  Saturation1/1 -> Change parameters from datasheet here/7(Eoff_igbt_nom)
  Switch/1 -> MATLAB Function3/1(T_m)  "torque"
  Divide1/1 -> idc/1  "idc"
  Voltage Measurement3/1 -> Memory2/1
  Change parameters from datasheet here/2(CPloss_diode) -> Add7/1, Gain8/1
  Add7/1 -> Controlled Current Source4/1
  Gain8/1 -> Add5/2, Mux1/2
  Change parameters from datasheet here/3(SPloss_igbt) -> Add6/2, Gain9/1
  Add3/1 -> Divide1/1, P_inv_total/1  "P_inv_total"
  Voltage Measurement2/1 -> Memory1/1
  Mux6/1 -> Scope11/1
  Saturation2/1 -> Change parameters from datasheet here/8(Erec_diode_nom)
  Saturation/1 -> Change parameters from datasheet here/6(Eon_igbt_nom)
  Change parameters from datasheet here/4(SPloss_diode) -> Add7/2, Gain10/1
  Gain9/1 -> Add5/3, Mux1/3
  Mux1/1 -> Scope10/1
  Gain7/1 -> Add5/1, Mux1/1
  Change parameters from datasheet here/1(CPloss_igbt) -> Gain7/1, Add6/1
  Constant4/1 -> Change parameters from datasheet here/4(fs)
  Memory1/1 -> Change parameters from datasheet here/9(T_igbt), Mux6/1, Eoff_igbt_nom/1, Eon_igbt_nom/1
  Memory2/1 -> Mux6/2, Erec_diode_nom/1, Change parameters from datasheet here/10(T_diode)
  Gain10/1 -> Mux1/4, Add5/4
  Constant1/1 -> P = 3*Up*Ip*costheta/1
  Add5/1 -> Add3/2, Conduction_and_Switching_loss/1  "P_inv_loss"
  Add6/1 -> Controlled Current Source3/1
  Mux2/1 -> Scope3/1
  udc/1 -> Divide1/2, Change parameters from datasheet here/2(udc)  "udc"
  MATLAB Function3/3(costheta) -> Mux2/3, P = 3*Up*Ip*costheta/4, Change parameters from datasheet here/5(costheta)
  Gain5/1 -> Change parameters from datasheet here/1(ic), Mux2/2, P = 3*Up*Ip*costheta/3
  MATLAB Function3/1(u) -> Gain4/1  "u"
  MATLAB Function3/2(i) -> Gain5/1  "i"
  MATLAB Function/1(u_sq) -> MATLAB Function3/2(usq)
  MATLAB Function/2(u_sd) -> MATLAB Function3/3(usd)
  Gain/1 -> MATLAB Function/3(w_mech)
  udc1/1 -> MATLAB Function/2(udc)  "udc"
  terminal_power/1 -> Add3/1, P_mot_elec/1
  Zero/1 -> Switch/3
  rpm/1 -> Switch/2, Product/3, MATLAB Function3/4(n), Gain/1
  Constant/1 -> Product/2
  Product/1 -> Switch/1
  terminal_power1/1 -> Product/1
  From Workspace/1 -> Zero-Order Hold/1
  Zero-Order Hold/1 -> MATLAB Function/1(t)
  connections:
  RC15/RConn1 -- RC12/LConn1
  RC17/LConn1 -- RC16/RConn1
  RC15/LConn1 -- RC16/LConn1
  RC20/LConn1 -- RC21/RConn1
  DC Voltage Source1/RConn1 -- RC19/LConn1
  RC13/LConn1 -- RC22/RConn1
  RC21/LConn1 -- RC22/LConn1
  RC17/RConn1 -- RC13/RConn1 -- RC19/RConn1
  Voltage Measurement2/LConn2 -- Voltage Measurement3/LConn2 -- Controlled Current Source4/LConn1 -- DC Voltage Source1/LConn1 -- Controlled Current Source3/LConn1
  RC12/RConn1 -- Controlled Current Source3/RConn1 -- Voltage Measurement2/LConn1 -- Voltage Measurement3/LConn1 -- RC20/RConn1 -- Controlled Current Source4/RConn1

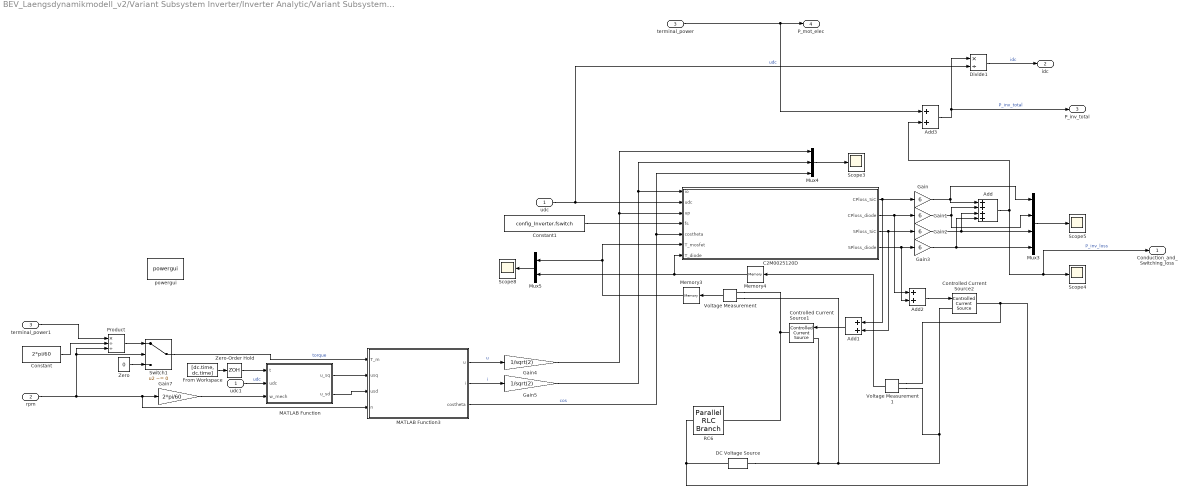
== system BEV_Laengsdynamikmodell_v2/Variant Subsystem Inverter/Inverter Analytic/Variant Subsystem/IM_Inverter_SiC-MOSFET_Analytic ==
  udc : Inport
  rpm : Inport  Port=2
  terminal_power : Inport  Port=3
  Add : Sum  Inputs=++++
  Add1 : Sum
  Add2 : Sum
  Add3 : Sum
  C2M0025120D : MATLAB Function  TreatAsAtomicUnit=on
  Constant : Constant  Value=2*pi/60
  Constant1 : Constant  Value=config_Inverter.fswitch
  Controlled Current Source1 : spsControlledCurrentSourceLib/Controlled Current Source  Initialize=on  Source_Type=AC  Amplitude=0  Phase=0  Frequency=0  Measurements=None
  Controlled Current Source2 : spsControlledCurrentSourceLib/Controlled Current Source  Initialize=on  Source_Type=AC  Amplitude=0  Phase=0  Frequency=0  Measurements=None
  DC Voltage Source : spsDCVoltageSourceLib/DC Voltage Source  Amplitude=25  Measurements=None
  Divide1 : Product  Inputs=*/
  From Workspace : FromWorkspace  VariableName=[dc.time, dc.time]
  Gain{,1..3} (4 alike) : Gain  Gain=6
  Gain4 : Gain  Gain=1/sqrt(2)
  Gain5 : Gain  Gain=1/sqrt(2)
  Gain7 : Gain  Gain=2*pi/60
  MATLAB Function : MATLAB Function  TreatAsAtomicUnit=on
  MATLAB Function3 : MATLAB Function  TreatAsAtomicUnit=on
  Memory3 : Memory  InitialCondition=25  InheritSampleTime=on
  Memory4 : Memory  InitialCondition=25  InheritSampleTime=on
  Mux3 : Mux
  Mux4 : Mux  Inputs=3
  Mux5 : Mux  Inputs=2
  Product : Product  Inputs=*//
  RC6 : spsParallelRLCBranchLib/Parallel RLC Branch  LConnTagsString=a  RConnTagsString=__new0  BranchType=R  Resistance=config_Inverter.Rmosfet  Inductance=1e-3  SetiL0=off  InitialCurrent=0  Capacitance=175  Setx0=on  InitialVoltage=0  Measurements=None
  Scope{3..5,8} (4 alike) : Scope
  Switch1 : Switch  Criteria=u2 ~= 0  SaturateOnIntegerOverflow=off  InputSameDT=off
  Voltage Measurement : spsVoltageMeasurementLib/Voltage Measurement  PhasorSimulation=off  OutputType=Complex  PSBequivalent=0
  Voltage Measurement1 : spsVoltageMeasurementLib/Voltage Measurement  PhasorSimulation=off  OutputType=Complex  PSBequivalent=0
  Zero : Constant  Value=0  OutDataTypeStr=Inherit: Inherit via back propagation
  Zero-Order Hold : ZeroOrderHold  SampleTime=-1
  powergui : spspowerguiLib/powergui  Priority=1  SimulationMode=Discrete  SampleTime=1  frequency=60  Iterations=50  frequencyindice=0  Pbase=100e6  ErrMax=1e-4  UnitsV=kV  UnitsW=MW  buscounter=0  FunctionMessages=on  echomessages=on  EnableUseOfTLC=off  CurrentSourceSwitches=off  DisableSnubberDevices=off  DisableRonSwitches=off  DisableVfSwitches=off  DisplayEquations=off  AutomaticDiscreteSolvers=off  SolverType=Backward Euler  Interpol=off  ExternalGateDelay=off  methode=off  Ts=100  x0status=blocks  SPID=off  SwTol=0  HookPort=off  NonlinearTolerance=1e-4  nMaxIteration=100  ContinueOnMaxIteration=off  RestoreLinks=warning  ResistiveCurrentMeasurement=off  Frange=[0:2:500]  Ylog=off  Xlog=on  ShowGrid=off  save=off  variable=ZData  structure=0  ZoomFFT=off  StartTime=0.0  cycles=1  DisplayStyle=1  fundamental=60  FreqAxis=off  MaxFrequency=1000  frequencyindicesteady=1  RmsSteady=1  display=off
  terminal_power1 : InportShadow  Port=3
  udc1 : InportShadow
  Conduction_and_Switching_loss : Outport
  idc : Outport  Port=2
  P_inv_total : Outport  Port=3
  P_mot_elec : Outport  Port=4
  wires:
  terminal_power/1 -> Add3/1, P_mot_elec/1
  Add3/1 -> Divide1/1, P_inv_total/1  "P_inv_total"
  Gain5/1 -> Mux4/2, C2M0025120D/1(io)
  Gain4/1 -> Mux4/1, C2M0025120D/3(up)
  udc/1 -> C2M0025120D/2(udc), Divide1/2  "udc"
  Divide1/1 -> idc/1  "idc"
  Add/1 -> Scope4/1, Conduction_and_Switching_loss/1, Add3/2  "P_inv_loss"
  MATLAB Function3/3(costheta) -> Mux4/3, C2M0025120D/5(costheta)  "cos"
  MATLAB Function3/2(i) -> Gain5/1  "i"
  Mux3/1 -> Scope5/1
  Mux4/1 -> Scope3/1
  Voltage Measurement/1 -> Memory3/1
  Mux5/1 -> Scope8/1
  C2M0025120D/2(CPloss_diode) -> Gain1/1, Add2/1
  Constant1/1 -> C2M0025120D/4(fs)
  C2M0025120D/3(SPloss_SiC) -> Gain2/1, Add1/2
  Voltage Measurement1/1 -> Memory4/1
  Add2/1 -> Controlled Current Source2/1
  Memory4/1 -> Mux5/2, C2M0025120D/7(T_diode)
  Add1/1 -> Controlled Current Source1/1
  Gain/1 -> Add/1, Mux3/1
  C2M0025120D/4(SPloss_diode) -> Gain3/1, Add2/2
  Gain1/1 -> Add/2, Mux3/2
  Gain2/1 -> Add/3, Mux3/3
  C2M0025120D/1(CPloss_SiC) -> Gain/1, Add1/1
  Memory3/1 -> C2M0025120D/6(T_mosfet), Mux5/1
  Gain3/1 -> Mux3/4, Add/4
  MATLAB Function/1(u_sq) -> MATLAB Function3/2(usq)
  MATLAB Function/2(u_sd) -> MATLAB Function3/3(usd)
  MATLAB Function3/1(u) -> Gain4/1  "u"
  terminal_power1/1 -> Product/1
  udc1/1 -> MATLAB Function/2(udc)  "udc"
  rpm/1 -> Switch1/2, Product/3, MATLAB Function3/4(n), Gain7/1
  Gain7/1 -> MATLAB Function/3(w_mech)
  Zero/1 -> Switch1/3
  Product/1 -> Switch1/1
  Constant/1 -> Product/2
  Switch1/1 -> MATLAB Function3/1(T_m)  "torque"
  From Workspace/1 -> Zero-Order Hold/1
  Zero-Order Hold/1 -> MATLAB Function/1(t)
  connections:
  RC6/RConn1 -- Controlled Current Source1/RConn1 -- Voltage Measurement/LConn1
  Controlled Current Source2/LConn1 -- Voltage Measurement/LConn2 -- Controlled Current Source1/LConn1 -- DC Voltage Source/LConn1 -- Voltage Measurement1/LConn2
  Voltage Measurement1/LConn1 -- Controlled Current Source2/RConn1 -- RC6/LConn1 -- DC Voltage Source/RConn1
